simulink model "TEST_LIDAR"  (R2022b)
settings: Solver=FixedStepAuto  StartTime=0.0  StopTime=inf  FixedStep=1e-3  RelTol=1e-3  EnableMultiTasking=on
model workspace (MAT data in the model file):
  SL_ROS_VariableLengthArrays_MaxSizes : object (value not decoded)
values from neighbouring files (symbols this model uses):
  data = theClient.GetLastFrameOfData()    [FuncMotive.m]
undefined symbols (not defined in the file or in its folder): angular, carstamp, CIRCUIT, CLTF_DAMP, CLTF_FREQ, CLTF_GAIN, CONTROL, CONTROL_INI, DiscIntNeverNeededParam, INPUT, linear, MCP3201, MD25, MODEL, MODEL_INI, mpcstate, MPU60X0, MPU9250, MSG, NAV_MPC_CONTROL, OUTPUT, RCRX, SAMPLING_TIME, SYSID_INPUT, VL6180X
libraries: raspberrypiCommlib x160, simulink x89, raspberrypiNetworklib x22, ros2lib x14, dspsigattribs x14, embedlinuxBasiclib x12, ctrlSharedLib x2, mpclib x1, vrlib x1, sldrtlib x1
(part 12 of 19)

== matlab function TEST_LIDAR/HARDWARE/SENSORS/WALL RANGE SENSOR/ANGLE AND DISTANCE COMPUTATION/YAW_ANGLE_DISTANCE_COMPUTATION ==
  data: FRONT_DISTANCE input; CONTROL output Bus: CONTROL_Bus; REAR_DISTANCE input; CONTROL_IN input
function CONTROL = WALL_ORIENTATION(FRONT_DISTANCE,REAR_DISTANCE,CONTROL_IN)

%% UPDATE BUS
CONTROL = CONTROL_IN;
%% PARAMETERS
RANGE_SENS_DIST = CONTROL.PARAM.RANGE_SENS_DIST;
%% MEASUREMENTS
CONTROL.INPUT.RANGE_WALL_ANG = atan2((REAR_DISTANCE-FRONT_DISTANCE)/1000,RANGE_SENS_DIST);
CONTROL.INPUT.RANGE_WALL_DIST = (FRONT_DISTANCE+REAR_DISTANCE)/2*cos(CONTROL.INPUT.RANGE_WALL_ANG)/1000;
CONTROL.INPUT.RANGE_FRONT_DIST = FRONT_DISTANCE/1000; % m
CONTROL.INPUT.RANGE_REAR_DIST = REAR_DISTANCE/1000; % m

return

== matlab function TEST_LIDAR/HARDWARE/SENSORS/IMU MPU60X0_SPI/READ IMU/IMU CALIBRATION ==
  data: CONTROL_IN input; ACCEL input; ACCEL_FILT input; ACCEL_MEAN input; ACCEL_MEAN_FILT input; GYRO input; GYRO_FILT input; GYRO_MEAN input; GYRO_MEAN_FILT input; ACCEL_CALIB input; ALFA_CALIB input; ACCEL_OFFS_IN input; GYRO_OFFS_IN input; CONTROL output Bus: CONTROL_Bus; ACCEL_OFFS_OUT output; GYRO_OFFS_OUT output; GRAVITY_VECTOR input
function [CONTROL,ACCEL_OFFS_OUT,GYRO_OFFS_OUT] = IMU_CALIBRATION(CONTROL_IN,...
                       ACCEL,ACCEL_FILT,ACCEL_MEAN,ACCEL_MEAN_FILT,...
                       GYRO,GYRO_FILT,GYRO_MEAN,GYRO_MEAN_FILT,...
                       ACCEL_CALIB,ALFA_CALIB,ACCEL_OFFS_IN,GYRO_OFFS_IN,GRAVITY_VECTOR)
                        
%--------------------------------------------------------------
% COPY CONTROL BUS
%--------------------------------------------------------------
CONTROL = CONTROL_IN;

%--------------------------------------------------------------
% IMU ORIENTATION
%--------------------------------------------------------------
% ACCEL = [0 0 1 ; 1 0 0 ; 0 1 0]*ACCEL;
% GYRO = [0 0 1 ; 1 0 0 ; 0 1 0]*GYRO;
ACCEL_MEAN = [0 0 1 ; 1 0 0 ; 0 1 0]*ACCEL_MEAN;
GYRO_MEAN = [0 0 1 ; 1 0 0 ; 0 1 0]*GYRO_MEAN;
% ACCEL_FILT = [0 0 1 ; 1 0 0 ; 0 1 0]*ACCEL_FILT;
% GYRO_FILT = [0 0 1 ; 1 0 0 ; 0 1 0]*GYRO_FILT;
ACCEL_MEAN_FILT = [0 0 1 ; 1 0 0 ; 0 1 0]*ACCEL_MEAN_FILT;
GYRO_MEAN_FILT = [0 0 1 ; 1 0 0 ; 0 1 0]*GYRO_MEAN_FILT;

%--------------------------------------------------------------
% CALIBRATION 
%--------------------------------------------------------------
if CONTROL.STATE.CURRENT_STATUS_SYS == 1  % CALIBRATION ENABLED
    if ACCEL_CALIB % ACCELEROMETER CALIBRATION ENABLED
        ACCEL_OFFS_OUT = ALFA_CALIB*ACCEL_OFFS_IN + (1-ALFA_CALIB)*(ACCEL_MEAN_FILT-GRAVITY_VECTOR);
    else
        ACCEL_OFFS_OUT = ACCEL_OFFS_IN;
    end
    GYRO_OFFS_OUT  = ALFA_CALIB*GYRO_OFFS_IN  + (1-ALFA_CALIB)*GYRO_MEAN_FILT;
else % END OF CALIBRATION
    ACCEL_OFFS_OUT = ACCEL_OFFS_IN;  
    GYRO_OFFS_OUT  = GYRO_OFFS_IN;
    % ACCEL = ACCEL - ACCEL_OFFS_OUT;
    % GYRO = GYRO - GYRO_OFFS_OUT;
    ACCEL_MEAN = ACCEL_MEAN - ACCEL_OFFS_OUT;
    GYRO_MEAN = GYRO_MEAN - GYRO_OFFS_OUT;
    % ACCEL_FILT = ACCEL_FILT - ACCEL_OFFS_OUT;
    % GYRO_FILT = GYRO_FILT - GYRO_OFFS_OUT;
    ACCEL_MEAN_FILT = ACCEL_MEAN_FILT - ACCEL_OFFS_OUT;
    GYRO_MEAN_FILT = GYRO_MEAN_FILT - GYRO_OFFS_OUT;
end

%--------------------------------------------------------------
% IMU BUS UPDATE
%--------------------------------------------------------------
% CONTROL.INPUT.IMU_ACCEL = ACCEL;
% CONTROL.INPUT.IMU_GYRO = GYRO;
CONTROL.INPUT.IMU_ACCEL_MEAN = ACCEL_MEAN;
CONTROL.INPUT.IMU_GYRO_MEAN = GYRO_MEAN;
% CONTROL.INPUT.IMU_ACCEL_FILT = ACCEL_FILT;
% CONTROL.INPUT.IMU_GYRO_FILT = GYRO_FILT;
CONTROL.INPUT.IMU_ACCEL_MEAN_FILT = ACCEL_MEAN_FILT;
CONTROL.INPUT.IMU_GYRO_MEAN_FILT = GYRO_MEAN_FILT;

return

== matlab function TEST_LIDAR/CONTROL/STATE ESTIMATOR ==
  data: CONTROL_IN input Bus: CONTROL_Bus; CONTROL output Bus: CONTROL_Bus
 function CONTROL = STATE_ESTIMATOR(CONTROL_IN)

%--------------------------------------------------------------
% COPY CONTROL BUS
%--------------------------------------------------------------
CONTROL = CONTROL_IN;

%--------------------------------------------------------------
% CONTROL_STATUS
%--------------------------------------------------------------
% / 0. INITIALIZATION     / 1. ESTIMATION    / 2. ACTIVE CONTROL
if CONTROL.STATE.CONTROL_STATUS == 0 % INITIALIZATION
    return
end 

%--------------------------------------------------------------
% STATE
%--------------------------------------------------------------
persistent initialize IMU_EULER_ANG_CF NAV_SVF_STATE NAV_EARTH_POS_PRV ...
           x_v x_w P_v P_w uc_prv ud_prv...
           accel_lpf vel_lpf yaw_rate_lpf yaw_ang_lpf
           
if isempty(initialize)
    IMU_EULER_ANG_CF = zeros(3,1);
    if CONTROL.STATE.VEHICLE_MODE
        IMU_EULER_ANG_CF(2) = CONTROL.INPUT.IMU_PITCH_ANG_INI;
        CONTROL.EKF_IMU.STATE(2) = CONTROL.INPUT.IMU_PITCH_ANG_INI;
    end
    NAV_SVF_STATE = zeros(2,3);
    NAV_EARTH_POS_PRV = CONTROL.INPUT.NAV_EARTH_POS;
    x_v = zeros(3,1);
    x_w = zeros(4,1);
    P_v = eye(3);
    P_w = eye(4);
    uc_prv = 0;
    ud_prv = 0;
    accel_lpf = 0;
    vel_lpf = 0;
    yaw_rate_lpf = 0;
    yaw_ang_lpf = 0; 
    initialize = 1;
    if CONTROL.STATE.WALL_FOLLOWER_MODE % LIDAR 2D
        CONTROL.EKF_WFL.STATE(2) = 0.25;
    else % RANGE
        CONTROL.EKF_WFL.STATE(2) = 0.1;
    end
end

%--------------------------------------------------------------
% PARAMETERS
%--------------------------------------------------------------
ts = CONTROL.PARAM.SAMPLING_TIME;
PITCH_OFFSET = CONTROL.PARAM.IMU_PITCH_OFFSET;
GRAVITY = CONTROL.PARAM.GRAVITY;
% First-order models
Kv = CONTROL.PARAM.VEL_GAIN; 
Tv = CONTROL.PARAM.VEL_TIME_CONSTANT; 
Tf = 1/2/pi/CONTROL.PARAM.ENC_FILT_FREQ;
% Distance between wheeels (m)
W = CONTROL.PARAM.WHEEL_DISTANCE;
% Wheel radius (m)
R = CONTROL.PARAM.WHEEL_RADIUS;
% Wheel gear ratio
WHEEL_GEAR_RATIO = CONTROL.PARAM.WHEEL_GEAR_RATIO;
% Encoder filter frequency (Hz)
ENC_FILT_FREQ = CONTROL.PARAM.ENC_FILT_FREQ;

%--------------------------------------------------------------
% UPDATE MEASUREMENTS
%--------------------------------------------------------------
% REAL MOTOR VOLTAGES (after applying the pwm rate limit)
uc = CONTROL.OUTPUT.REAL_MOTOR_VOLT_CD(1);
ud = CONTROL.OUTPUT.REAL_MOTOR_VOLT_CD(2);
% ENCODER ANGLES
inc2_com_ang = CONTROL.INPUT.ENC_INC2_COM_ANG;
inc_com_ang = CONTROL.INPUT.ENC_INC_COM_ANG;
inc_dif_ang = CONTROL.INPUT.ENC_INC_DIF_ANG;
dif_ang = CONTROL.INPUT.ENC_DIF_ANG;
ENC_YAW_ANG_KF = CONTROL.INPUT.ENC_YAW_ANG_KF;
% IMU
IMU_ACCEL_MEAN_CAR = CONTROL.INPUT.IMU_ACCEL_MEAN;
IMU_ACCEL_MEAN_FILT_CAR = CONTROL.INPUT.IMU_ACCEL_MEAN_FILT;
IMU_GYRO_MEAN_CAR = CONTROL.INPUT.IMU_GYRO_MEAN;
IMU_GYRO_MEAN_FILT_CAR = CONTROL.INPUT.IMU_GYRO_MEAN_FILT;
% NAVIGATION SYSTEM (CAR MODE)
if CONTROL.STATE.NAV_MODE==1 % (MCS)
    CONTROL.INPUT.NAV_EARTH_POS = CONTROL.INPUT.MCS_EARTH_POS;
    CONTROL.INPUT.NAV_EULER_ANG = CONTROL.INPUT.MCS_EULER_ANG;
end 
NAV_EARTH_POS = CONTROL.INPUT.NAV_EARTH_POS;
NAV_EULER_ANG_CAR = CONTROL.INPUT.NAV_EULER_ANG; 
 
%--------------------------------------------------------------
% IMU ORIENTATION (SELF-BALANCING VEHICLE)
%--------------------------------------------------------------
if CONTROL.STATE.VEHICLE_MODE 
    % CAR REFERENCE FRAME -> SBV REFERENCE FRAME
    ROTATION_MATRIX = [cos(PITCH_OFFSET) 0 -sin(PITCH_OFFSET)
                              0         1          0
                      sin(PITCH_OFFSET) 0 cos(PITCH_OFFSET)]*...
                      [0 0 1 ; 0 1 0 ; -1 0 0];
    IMU_ACCEL_MEAN_SBV = ROTATION_MATRIX*IMU_ACCEL_MEAN_CAR;
    IMU_ACCEL_MEAN_FILT_SBV = ROTATION_MATRIX*IMU_ACCEL_MEAN_FILT_CAR;
    IMU_GYRO_MEAN_SBV = ROTATION_MATRIX*IMU_GYRO_MEAN_CAR;
    IMU_GYRO_MEAN_FILT_SBV = ROTATION_MATRIX*IMU_GYRO_MEAN_FILT_CAR;    
    % Rotation matrix (ZYX): CAR REFERENCE FRAME ->  EARTH REFERENCE FRAME
    % s_x1 = sin(NAV_EULER_ANG_CAR(1));
    % c_x1 = cos(NAV_EULER_ANG_CAR(1));
    % s_x2 = sin(NAV_EULER_ANG_CAR(2));
    % c_x2 = cos(NAV_EULER_ANG_CAR(2));
    % s_x3 = sin(NAV_EULER_ANG_CAR(3));
    % c_x3 = cos(NAV_EULER_ANG_CAR(3));
    % matDCM_BE = [ cos(Theta)*cos(Shi) sin(Phi)*sin(Theta)*cos(Shi)-cos(Phi)*sin(Shi)  cos(Phi)*sin(Theta)*cos(Shi)+sin(Phi)*sin(Shi)
    %               cos(Theta)*sin(Shi) sin(Phi)*sin(Theta)*sin(Shi)+cos(Phi)*cos(Shi)  cos(Phi)*sin(Theta)*sin(Shi)-sin(Phi)*cos(Shi)
    %                    -sin(Theta)          sin(Phi)*cos(Theta)                             cos(Phi)*cos(Theta)                           ];
    % matDCM_BE_CAR =     [         c_x2*c_x3         s_x1*s_x2*c_x3-c_x1*s_x3      c_x1*s_x2*c_x3+s_x1*s_x3
    %                              c_x2*s_x3         s_x1*s_x2*s_x3+c_x1*c_x3      c_x1*s_x2*s_x3-s_x1*c_x3
    %                               -s_x2                   s_x1*c_x2                      c_x1*c_x2     ];
    % matDCM_BE_CAR = matDCM_BE_SBV*ROTATION_MATRIX
    % matDCM_BE_SBV = matDCM_BE_CAR/ROTATION_MATRIX;
    % NAV_EULER_ANG_SBV = zeros(1,3);
    % NAV_EULER_ANG_SBV(1:3) = rotm2eul(matDCM_BE_SBV,'ZYX');
    % NAV_EULER_ANG_SBV = ROTATION_MATRIX*NAV_EULER_ANG_CAR;
    NAV_EULER_ANG_SBV = zeros(3,1);
    NAV_EULER_ANG_SBV(1) = 0;
    NAV_EULER_ANG_SBV(2) = NAV_EULER_ANG_CAR(2)-pi/2+PITCH_OFFSET;
    NAV_EULER_ANG_SBV(3) = -NAV_EULER_ANG_CAR(1);
    NAV_EULER_ANG = NAV_EULER_ANG_SBV(:);
    IMU_ACCEL_MEAN_FILT = IMU_ACCEL_MEAN_FILT_SBV;
    IMU_GYRO_MEAN_FILT = IMU_GYRO_MEAN_FILT_SBV;
    IMU_ACCEL_MEAN = IMU_ACCEL_MEAN_SBV;
    IMU_GYRO_MEAN = IMU_GYRO_MEAN_SBV;
else
    NAV_EULER_ANG = NAV_EULER_ANG_CAR;
    IMU_ACCEL_MEAN_FILT = IMU_ACCEL_MEAN_FILT_CAR;
    IMU_GYRO_MEAN_FILT = IMU_GYRO_MEAN_FILT_CAR;
    IMU_ACCEL_MEAN = IMU_ACCEL_MEAN_CAR;
    IMU_GYRO_MEAN = IMU_GYRO_MEAN_CAR;
end

%--------------------------------------------------------------
% COMPLEMENTARY FILTER
%--------------------------------------------------------------
IMU_CF_ALFA = exp(-ts*2*pi*CONTROL.PARAM.IMU_CF_FREQ);
IMU_ACCEL_CF = IMU_ACCEL_MEAN_FILT;
% IMU_ACCEL_CF = IMU_ACCEL_MEAN;
% s_x1 = sin(IMU_EULER_ANG_CF(1));
% c_x1 = cos(IMU_EULER_ANG_CF(1));
% c_x2 = cos(IMU_EULER_ANG_CF(2));
% t_x2 = tan(IMU_EULER_ANG_CF(2));
% dEuler = inv_matEuler*wxyz;
% inv_matEuler = [ 1       s_x1*t_x2      c_x1*t_x2
%                  0          c_x1          -s_x1
%                  0       s_x1/c_x2      c_x1/c_x2     ];
% IMU_EULER_RATE_CF = inv_matEuler*IMU_GYRO_MEAN_FILT;
% IMU_EULER_RATE_CF = inv_matEuler*IMU_GYRO_MEAN;
IMU_EULER_RATE_CF = IMU_GYRO_MEAN_FILT;
% IMU_EULER_RATE_CF = IMU_GYRO_MEAN;
% ax =  g*sin(x2)           ->  x2 = asin(ax/g)
% ay = -g*sin(x1)*cos(x2)   ->  x1 = asin(-ay/g/cos(x2))
% az = -g*cos(x1)*cos(x2)
% if abs(IMU_ACCEL_MEAN_FILT(1)) < 0.9*GRAVITY
%     IMU_EULER_ANG_CF(2) = (IMU_EULER_ANG_CF(2) + IMU_EULER_RATE_CF(2)*ts)*IMU_CF_ALFA + ...
%         asin(IMU_ACCEL_CF(1)/GRAVITY)*(1-IMU_CF_ALFA);
% else
%     IMU_EULER_ANG_CF(2) = IMU_EULER_ANG_CF(2) + IMU_EULER_RATE_CF(2)*ts;
% end
% if abs(IMU_ACCEL_CF(2)) < 0.9*GRAVITY*cos(IMU_EULER_ANG_CF(2))
%     IMU_EULER_ANG_CF(1) = (IMU_EULER_ANG_CF(1) + IMU_EULER_RATE_CF(1)*ts)*IMU_CF_ALFA + ...
%         asin(-IMU_ACCEL_CF(2)/GRAVITY/cos(IMU_EULER_ANG_CF(2)))*(1-IMU_CF_ALFA);
% else
%     IMU_EULER_ANG_CF(1) = IMU_EULER_ANG_CF(1) + IMU_EULER_RATE_CF(1)*ts;
% end
% IMU_EULER_ANG_CF = NAV_EULER_ANG;
IMU_EULER_ANG_CF(1) = (IMU_EULER_ANG_CF(1) + IMU_EULER_RATE_CF(1)*ts)*IMU_CF_ALFA + ...
    atan2(-IMU_ACCEL_CF(2),-IMU_ACCEL_CF(3))*(1-IMU_CF_ALFA);
IMU_EULER_ANG_CF(2) = (IMU_EULER_ANG_CF(2) + IMU_EULER_RATE_CF(2)*ts)*IMU_CF_ALFA + ...
    atan2(IMU_ACCEL_CF(1),-IMU_ACCEL_CF(3))*(1-IMU_CF_ALFA);
IMU_EULER_ANG_CF(3) = (IMU_EULER_ANG_CF(3) + IMU_EULER_RATE_CF(3)*ts);
CONTROL.INPUT.IMU_EULER_ANG_CF = IMU_EULER_ANG_CF;
% CONTROL.INPUT.IMU_EULER_RATE_CF = IMU_EULER_RATE_CF;
CONTROL.INPUT.IMU_EULER_RATE_CF = IMU_EULER_RATE_CF;
IMU_FORWARD_ACCEL_CF = IMU_ACCEL_CF(1) - GRAVITY*sin(IMU_EULER_ANG_CF(2));
CONTROL.INPUT.IMU_FORWARD_ACCEL_CF = IMU_FORWARD_ACCEL_CF;

%--------------------------------------------------------------
% NAVIGATION FILTER
%--------------------------------------------------------------
% x[k] = Ad*x[k-1] + B1d*u[k-1] + B2d*u[k]
% y[k] = Cd*x[k]   + Dd*u[k] 
Ad = CONTROL.PARAM.SVF_Ad;
B1d = CONTROL.PARAM.SVF_B1d;
B2d = CONTROL.PARAM.SVF_B2d;
Cd = CONTROL.PARAM.SVF_Cd;
Dd = CONTROL.PARAM.SVF_Dd;
NAV_EARTH_POS_FILT = zeros(3,1);
NAV_EARTH_VEL_FILT = zeros(3,1);
NAV_EARTH_ACCEL_FILT = zeros(3,1);
for nn = 1:3
    NAV_SVF_STATE(:,nn) = Ad*NAV_SVF_STATE(:,nn) + ...
                          B1d*NAV_EARTH_POS_PRV(nn) + B2d*NAV_EARTH_POS(nn);
    aux = Cd*NAV_SVF_STATE(:,nn) + Dd*NAV_EARTH_POS(nn);
    NAV_EARTH_POS_FILT(nn) = aux(1);
    NAV_EARTH_VEL_FILT(nn) = aux(2);  
    NAV_EARTH_ACCEL_FILT(nn) = aux(3);
end
NAV_EARTH_POS_PRV = NAV_EARTH_POS;
CONTROL.INPUT.NAV_EARTH_POS_FILT = NAV_EARTH_POS_FILT;
CONTROL.INPUT.NAV_EARTH_VEL_FILT = NAV_EARTH_VEL_FILT;
CONTROL.INPUT.NAV_EARTH_ACCEL_FILT = NAV_EARTH_ACCEL_FILT;

%--------------------------------------------------------------
% IMU EKF UPDATE
%--------------------------------------------------------------
% EKF INPUT = GYRO_MEAN
CONTROL.EKF_IMU.INPUT = IMU_GYRO_MEAN_FILT;
% EKF OBSRV = [ACCEL ; ENC_YAW_ANG ; NAV_EULER_ANG];
CONTROL.EKF_IMU.OBSRV = [IMU_ACCEL_MEAN_FILT ; x_w(4) ; NAV_EULER_ANG];
CONTROL.EKF_IMU.ESTIMATION_MODE = CONTROL.STATE.NAV_MODE + uint8(1);
% EKF UPDATE
CONTROL.EKF_IMU = EKF_IMU(CONTROL.EKF_IMU);
% EKF STATE = [EULER_ANG ; GYRO_BIAS];
CONTROL.INPUT.IMU_EULER_ANG_KF = CONTROL.EKF_IMU.STATE(1:3);
CONTROL.INPUT.IMU_EULER_RATE_KF = IMU_GYRO_MEAN_FILT - CONTROL.EKF_IMU.STATE(4:6);
% IMU forward acceleration 
IMU_FORWARD_ACCEL_KF = IMU_ACCEL_MEAN_FILT(1) - GRAVITY*sin(CONTROL.INPUT.IMU_EULER_ANG_KF(2));
CONTROL.INPUT.IMU_FORWARD_ACCEL_KF = IMU_FORWARD_ACCEL_KF;   

%--------------------------------------------------------------
% ENCODER FILTERING: LOW-PASS FILTER
%--------------------------------------------------------------
% LPF discrete-time pole
ALFA = exp(-ts*2*pi*ENC_FILT_FREQ);
% Low-pass filtering
accel_lpf = ALFA*accel_lpf + (1-ALFA)*pi/180*R*inc2_com_ang/ts^2;
vel_lpf = ALFA*vel_lpf + (1-ALFA)*pi/180*R*inc_com_ang/ts;
yaw_rate_lpf = ALFA*yaw_rate_lpf + (1-ALFA)*pi/180*2*R/W*inc_dif_ang/ts;
yaw_ang_lpf = ALFA*yaw_ang_lpf + (1-ALFA)*pi/180*2*R/W*dif_ang;

%--------------------------------------------------------------
% ENCODER FILTERING: KALMAN FILTER
%--------------------------------------------------------------
% MODEL: Process   
% x[k] = Ad*x[k-1] + Bd*u[k-1] + w[k]
% MODEL: Measurement 
% z[k] = Cd*x[k] + v[k]
%---------------------------------------------------------
% KF: Prediction stage
% x[k|k-1] = Ad*x[k-1|k-1] + B1d*u[k-1] + B2d*u[k]
% P[k|k-1] = Ad*P[k-1|k-1]*Ad' + Q[k]
% KF: Update stage
% e = z[k] - Cd*x[k|k-1]
% S[k] = Cd*P[k|k-1]*Cd' + R[k]
% K[k] = P[k|k-1]*Cd'*inv(S[k])
% x[k|k] = x[k|k-1] + K[k]*e[k]
% P[k|k] = (I - K[k]Cd)*P[k|k-1]
%---------------------------------------------------------
Ad_v = CONTROL.PARAM.ENC_FORWARD_VEL_matAd;
Bd_v = CONTROL.PARAM.ENC_FORWARD_VEL_matBd;
Cd_v = CONTROL.PARAM.ENC_FORWARD_VEL_matCd;
Q_v = diag(CONTROL.PARAM.ENC_FORWARD_VEL_matQ);
R_v = diag(CONTROL.PARAM.ENC_FORWARD_VEL_matR);
x_v = Ad_v*x_v + Bd_v*uc_prv;
P_v = Ad_v*P_v*Ad_v' + Q_v;
e_v = [vel_lpf ; IMU_FORWARD_ACCEL_KF] - Cd_v*x_v;
S_v = Cd_v*P_v*Cd_v' + R_v;
K_v = P_v*Cd_v'/S_v;
x_v = x_v + K_v*e_v;
P_v = (eye(3) - K_v*Cd_v)*P_v;
uc_prv = uc;
%---------------------------------------------------------
Ad_w = CONTROL.PARAM.ENC_YAW_RATE_matAd;
Bd_w = CONTROL.PARAM.ENC_YAW_RATE_matBd;
Cd_w = CONTROL.PARAM.ENC_YAW_RATE_matCd;
Q_w = diag(CONTROL.PARAM.ENC_YAW_RATE_matQ);
R_w = diag(CONTROL.PARAM.ENC_YAW_RATE_matR);
x_w = Ad_w*x_w + Bd_w*ud_prv;
P_w = Ad_w*P_w*Ad_w' + Q_w;
e_w = [yaw_rate_lpf ; IMU_GYRO_MEAN_FILT(3)] - Cd_w*x_w;
S_w = Cd_w*P_w*Cd_w' + R_w;
K_w = P_w*Cd_w'/S_w;
x_w = x_w + K_w*e_w;
P_w = (eye(4) - K_w*Cd_w)*P_w;
ud_prv = ud;

%--------------------------------------------------------------
% ENCODER FORWARD VELOCITY
%--------------------------------------------------------------
CONTROL.INPUT.ENC_FORWARD_ACCEL_LPF = accel_lpf;
CONTROL.INPUT.ENC_FORWARD_VEL_LPF = vel_lpf;
CONTROL.INPUT.ENC_FORWARD_ACCEL_KF = -1/Tf*x_v(3) + 1/Tf*x_v(1);
CONTROL.INPUT.ENC_FORWARD_VEL_KF = x_v(3);

%--------------------------------------------------------------
% ENCODER YAW RATE
%--------------------------------------------------------------
CONTROL.INPUT.ENC_YAW_RATE_LPF = yaw_rate_lpf;
CONTROL.INPUT.ENC_YAW_RATE_KF = x_w(3);

%--------------------------------------------------------------
% ENCODER YAW ANGLE UNWRAPPING
%--------------------------------------------------------------
aux1 = pi/180*2*R/W*dif_ang;
aux2 = CONTROL.TARGET.YAW_ANG_REF;
INC_YAW_ANG = [aux1-aux2
               aux1-aux2-2*pi
               aux1-aux2+2*pi];
[~,ind] = min(abs(INC_YAW_ANG));
CONTROL.INPUT.ENC_YAW_ANG = aux2 + INC_YAW_ANG(ind);
aux1 = yaw_ang_lpf;
INC_YAW_ANG = [aux1-aux2
               aux1-aux2-2*pi
               aux1-aux2+2*pi];
[~,ind] = min(abs(INC_YAW_ANG));
CONTROL.INPUT.ENC_YAW_ANG_LPF = aux2 + INC_YAW_ANG(ind);
aux1 = x_w(4);
INC_YAW_ANG = [aux1-aux2
               aux1-aux2-2*pi
               aux1-aux2+2*pi];
[~,ind] = min(abs(INC_YAW_ANG));
CONTROL.INPUT.ENC_YAW_ANG_KF = aux2 + INC_YAW_ANG(ind);

%--------------------------------------------------------------
% ENCODER MOTOR RATE
%--------------------------------------------------------------
CONTROL.INPUT.ENC_MOTOR_RATE_CD_LPF(1) = WHEEL_GEAR_RATIO*vel_lpf/R;
CONTROL.INPUT.ENC_MOTOR_RATE_CD_KF(1) = WHEEL_GEAR_RATIO*x_v(3)/R;
CONTROL.INPUT.ENC_MOTOR_RATE_CD_LPF(2) = WHEEL_GEAR_RATIO*W/R/2*yaw_rate_lpf;
CONTROL.INPUT.ENC_MOTOR_RATE_CD_KF(2) = WHEEL_GEAR_RATIO*W/R/2*x_w(3);
CONTROL.INPUT.ENC_MOTOR_RATE_LPF(1) = sum(CONTROL.INPUT.ENC_MOTOR_RATE_CD_LPF);
CONTROL.INPUT.ENC_MOTOR_RATE_KF(1) = sum(CONTROL.INPUT.ENC_MOTOR_RATE_CD_KF);
CONTROL.INPUT.ENC_MOTOR_RATE_LPF(2) = -diff(CONTROL.INPUT.ENC_MOTOR_RATE_CD_LPF);
CONTROL.INPUT.ENC_MOTOR_RATE_KF(2) = -diff(CONTROL.INPUT.ENC_MOTOR_RATE_CD_KF);

%--------------------------------------------------------------------------
% WALL FOLLOWER: DISTANCE AND ANGLE ESTIMATION USING THE LIDAR 2D
%--------------------------------------------------------------------------
if (CONTROL.STATE.CONTROL_MODE==4 || CONTROL.STATE.CONTROL_MODE==5) && ...
    CONTROL.STATE.WALL_FOLLOWER_MODE==1
    % The Lidar 2D 0 deg axis coincides with the vehicle negative X axis
    % The Lidar 2D rotates clockwise
    LIDAR_2D_ANG = CONTROL.EKF_WFL.PARAM.LIDAR_2D_WFL_ANG_SIGN*CONTROL.INPUT.LIDAR_2D(:,1) + ...
        CONTROL.EKF_WFL.PARAM.LIDAR_2D_WFL_ANG_OFFS;
    LIDAR_2D_DIST = CONTROL.INPUT.LIDAR_2D(:,2);
    ind = LIDAR_2D_ANG<=60 & LIDAR_2D_ANG>=-30 & ...
          LIDAR_2D_DIST>=0.1 & LIDAR_2D_DIST<=0.4;   
    N = sum(ind);
    % d = dm*cos(alfa-theta) = dm*cos(alfa)*cos(theta) + dm*sin(alfa)*sin(theta)
    % Least squares to estimate cos(theta)/d and sin(theta)/d
    % 1 = [dm*cos(alfa) dm*sin(alfa)]*[cos(theta)/d sin(theta)/d]'
    if N>=5 && abs(max(LIDAR_2D_ANG(ind))-min(LIDAR_2D_ANG(ind)))>=22.5
        % B = A*param
        B = ones(N,1);
        A = [LIDAR_2D_DIST(ind).*cosd(LIDAR_2D_ANG(ind)) LIDAR_2D_DIST(ind).*sind(LIDAR_2D_ANG(ind))];
        param = A\B;
        CONTROL.INPUT.LIDAR_2D_WALL_DIST = 1/sqrt(param(1)^2+param(2)^2);
        if abs(CONTROL.INPUT.LIDAR_2D_WALL_DIST*param(2))<1
            CONTROL.INPUT.LIDAR_2D_WALL_ANG = pi/180*asind(CONTROL.INPUT.LIDAR_2D_WALL_DIST*param(2));
        end
    end
end

%--------------------------------------------------------------------------
% WALL FOLLOWER FILTERING
%--------------------------------------------------------------------------
if CONTROL.STATE.CONTROL_MODE==4 || CONTROL.STATE.CONTROL_MODE==5
    % FILTER
    ALFA = exp(-CONTROL.PARAM.SAMPLING_TIME*2*pi*CONTROL_IN.PARAM.WFL_FILT_FREQ);
    if CONTROL.STATE.WALL_FOLLOWER_MODE==0 % RANGE SENSOR
        CONTROL.INPUT.WALL_ANG_FILT = ALFA*CONTROL.INPUT.WALL_ANG_FILT + (1-ALFA)*CONTROL.INPUT.RANGE_WALL_ANG;
        CONTROL.INPUT.WALL_DIST_FILT = ALFA*CONTROL.INPUT.WALL_DIST_FILT + (1-ALFA)*CONTROL.INPUT.RANGE_WALL_DIST;
    else % LIDAR 2D
        CONTROL.INPUT.WALL_ANG_FILT = ALFA*CONTROL.INPUT.WALL_ANG_FILT + (1-ALFA)*CONTROL.INPUT.LIDAR_2D_WALL_ANG;
        CONTROL.INPUT.WALL_DIST_FILT = ALFA*CONTROL.INPUT.WALL_DIST_FILT + (1-ALFA)*CONTROL.INPUT.LIDAR_2D_WALL_DIST;
    end
end

%--------------------------------------------------------------
% WALL FOLLOWER EKF UPDATE
%--------------------------------------------------------------
if CONTROL.STATE.CONTROL_MODE==4 || CONTROL.STATE.CONTROL_MODE==5    
    CONTROL.EKF_WFL.ESTIMATION_MODE = uint8(1);
    % EKF INPUT = [FORWARD_VEL ; YAW_RATE]
    CONTROL.EKF_WFL.INPUT = [CONTROL.INPUT.ENC_FORWARD_VEL_KF
                             CONTROL.INPUT.ENC_YAW_RATE_KF];
    % EKF OBSRV = [WALL_ANG ; WALL_DIST]
    CONTROL.EKF_WFL.PARAM.WALL_FOLLOWER_MODE = CONTROL.STATE.WALL_FOLLOWER_MODE;
    if CONTROL.STATE.WALL_FOLLOWER_MODE==0 % RANGE SENSOR
        CONTROL.EKF_WFL.OBSRV = [CONTROL.INPUT.RANGE_WALL_ANG ; CONTROL.INPUT.RANGE_WALL_DIST];
    else % LIDAR 2D
        CONTROL.EKF_WFL.OBSRV = [CONTROL.INPUT.LIDAR_2D_WALL_ANG ; CONTROL.INPUT.LIDAR_2D_WALL_DIST];
    end
    % EKF UPDATE
    CONTROL.EKF_WFL = EKF_WFL(CONTROL.EKF_WFL);
    % EKF STATE = [WALL_ANG ; WALL_DIST ; YAW_RATE_BIAS]
    CONTROL.INPUT.WALL_ANG_KF = CONTROL.EKF_WFL.STATE(1);
    CONTROL.INPUT.WALL_DIST_KF = CONTROL.EKF_WFL.STATE(2);
end

%--------------------------------------------------------------
% NAVIGATION EKF UPDATE
%--------------------------------------------------------------
if CONTROL.STATE.CONTROL_MODE==1 || CONTROL.STATE.CONTROL_MODE==3 ...
             || CONTROL.STATE.CONTROL_MODE==6
    % EKF INPUT = [FORWARD_VEL ; YAW_RATE]
    CONTROL.EKF_NAV.INPUT = [CONTROL.INPUT.ENC_FORWARD_VEL_KF
                             CONTROL.INPUT.ENC_YAW_RATE_KF];
    % EKF OBSRV = [NAV_YAW_ANG ; NAV_EARTH_POS_X ; NAV_EARTH_POS_Y]
    CONTROL.EKF_NAV.OBSRV = [NAV_EULER_ANG(3) ; NAV_EARTH_POS_FILT(1:2)];
    CONTROL.EKF_NAV.ESTIMATION_MODE = uint8(1);
    % EKF UPDATE
    CONTROL.EKF_NAV = EKF_NAV(CONTROL.EKF_NAV);
    % EKF STATE = [YAW_ANG ; EARTH_POS_X ; EARTH_POS_Y]
    CONTROL.INPUT.NAV_EULER_ANG_KF(3) = CONTROL.EKF_NAV.STATE(1);
    CONTROL.INPUT.NAV_EARTH_POS_KF(1:2) = CONTROL.EKF_NAV.STATE(2:3);
    CONTROL.INPUT.NAV_EARTH_POS_KF(3) = NAV_EARTH_POS_FILT(3);
end

%--------------------------------------------------------------
% STATE ESTIMATION
%--------------------------------------------------------------
if CONTROL.STATE.OBSERVER_MODE==1    
    %--------------------------------------------
    % EKF
    %--------------------------------------------
    CONTROL.INPUT.FORWARD_VEL = CONTROL.INPUT.ENC_FORWARD_VEL_KF;
    CONTROL.INPUT.PITCH_RATE = CONTROL.INPUT.IMU_EULER_RATE_KF(2);
    CONTROL.INPUT.PITCH_ANG = CONTROL.INPUT.IMU_EULER_ANG_KF(2);
    CONTROL.INPUT.YAW_RATE = CONTROL.INPUT.ENC_YAW_RATE_KF;
    if CONTROL.STATE.CONTROL_MODE==4 || CONTROL.STATE.CONTROL_MODE==5
        CONTROL.INPUT.YAW_ANG = CONTROL.INPUT.WALL_ANG_KF;
    elseif CONTROL.STATE.CONTROL_MODE==1 || CONTROL.STATE.CONTROL_MODE==3 ...
             || CONTROL.STATE.CONTROL_MODE==6    
        CONTROL.INPUT.YAW_ANG = CONTROL.INPUT.NAV_EULER_ANG_KF(3);
    else
        CONTROL.INPUT.YAW_ANG = ENC_YAW_ANG_KF;
    end    
    CONTROL.INPUT.WALL_DIST = CONTROL.INPUT.WALL_DIST_KF;
    CONTROL.INPUT.EARTH_POS = CONTROL.INPUT.NAV_EARTH_POS_KF;
    CONTROL.INPUT.MOTOR_RATE = CONTROL.INPUT.ENC_MOTOR_RATE_KF;
    CONTROL.INPUT.MOTOR_RATE_CD = CONTROL.INPUT.ENC_MOTOR_RATE_CD_KF;    
else
    %--------------------------------------------
    % FILTERED MEASUREMENT
    %--------------------------------------------
    CONTROL.INPUT.FORWARD_VEL = CONTROL.INPUT.ENC_FORWARD_VEL_LPF;
    CONTROL.INPUT.PITCH_RATE = CONTROL.INPUT.IMU_EULER_RATE_CF(2);
    CONTROL.INPUT.PITCH_ANG = CONTROL.INPUT.IMU_EULER_ANG_CF(2);
    % CONTROL.INPUT.PITCH_ANG = NAV_EULER_ANG(2);
    if CONTROL.STATE.ROTATION_MSRT_MODE % ENCODER
        CONTROL.INPUT.YAW_RATE = CONTROL.INPUT.ENC_YAW_RATE_LPF;
    else % IMU
        CONTROL.INPUT.YAW_RATE = CONTROL.INPUT.IMU_EULER_RATE_CF(3);
    end        
    if CONTROL.STATE.CONTROL_MODE==4 || CONTROL.STATE.CONTROL_MODE==5
        CONTROL.INPUT.YAW_ANG = CONTROL.INPUT.WALL_ANG_FILT;
    elseif CONTROL.STATE.CONTROL_MODE==1 || CONTROL.STATE.CONTROL_MODE==3 ...
             || CONTROL.STATE.CONTROL_MODE==6    
        CONTROL.INPUT.YAW_ANG = NAV_EULER_ANG(3);
    else
        CONTROL.INPUT.YAW_ANG = CONTROL.INPUT.ENC_YAW_ANG_LPF;
    end
    CONTROL.INPUT.WALL_DIST = CONTROL.INPUT.WALL_DIST_FILT;
    CONTROL.INPUT.EARTH_POS = NAV_EARTH_POS_FILT;
    CONTROL.INPUT.MOTOR_RATE = CONTROL.INPUT.ENC_MOTOR_RATE_LPF;
    CONTROL.INPUT.MOTOR_RATE_CD = CONTROL.INPUT.ENC_MOTOR_RATE_CD_LPF;
end
if CONTROL.STATE.NAV_TARGET_REACHED==1
    CONTROL.INPUT.FORWARD_VEL = 0;
    CONTROL.INPUT.YAW_RATE = 0;
end
CONTROL.INPUT.EARTH_VEL = NAV_EARTH_VEL_FILT;
CONTROL.INPUT.STATE = [CONTROL.INPUT.FORWARD_VEL ; CONTROL.INPUT.YAW_RATE ; ...
                       CONTROL.INPUT.YAW_ANG ; CONTROL.INPUT.WALL_DIST ; ...                      
                       CONTROL.INPUT.PITCH_RATE ; CONTROL.INPUT.PITCH_ANG];
CONTROL.INPUT.NAV_MO = CONTROL.INPUT.EARTH_POS(1:2);
return
